simulink model "arinc429_decoder"  (R2021a)
settings: Solver=VariableStepAuto  StartTime=0.0  StopTime=32e-5  RelTol=1e-3
libraries: fl_lib x72, ee_lib x26, nesl_utility x10
(part 1 of 2)
settings Model: Creator=sbetu  LastModifiedBy=sbetu

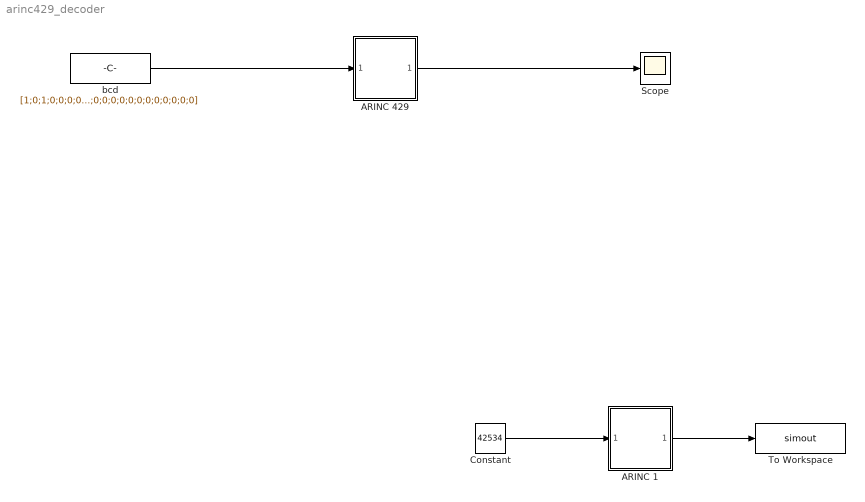
== system arinc429_decoder ==
  ARINC 1 : Subsystem
  ARINC 429 : Subsystem
  Constant : Constant  Value=42534  OutDataTypeStr=double
  Scope : Scope
  To Workspace : ToWorkspace  VariableName=simout  SampleTime=-1
  bcd : Constant  Value=[1;0;1;0;0;0;0;0;0;0;0;0;0;0;0;0;0;0;0]  VectorParams1D=off
  wires:
  bcd/1 -> ARINC 429/1(data 11-29)
  ARINC 429/1(Outport) -> Scope/1
  ARINC 1/1(Outport) -> To Workspace/1
  Constant/1 -> ARINC 1/1(data 11-29)

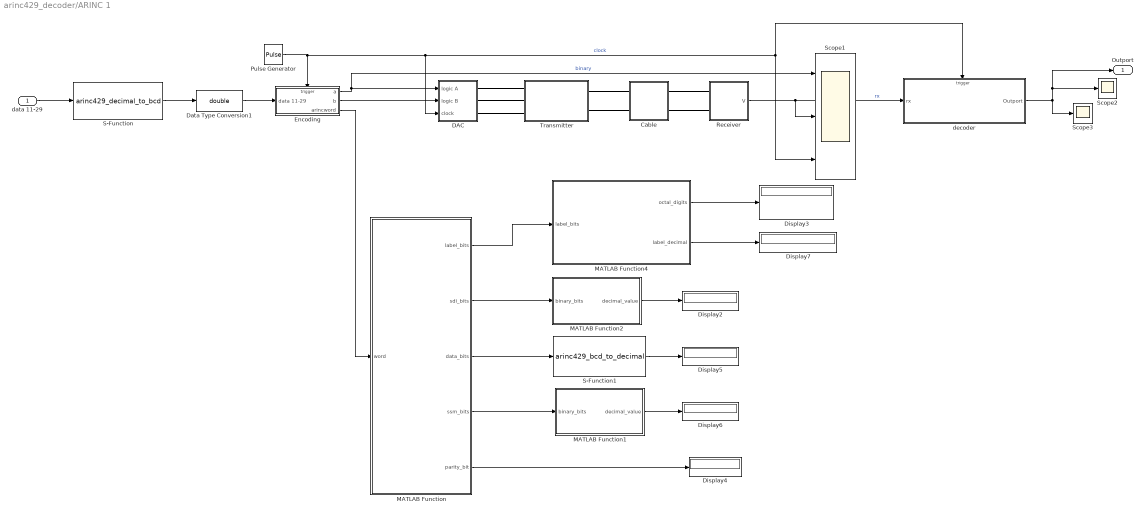
== system arinc429_decoder/ARINC 1 ==
  data 11-29 : Inport
  Cable : Subsystem
  DAC : Subsystem
  Data Type Conversion1 : DataTypeConversion  OutDataTypeStr=double
  Display{2..7} (6 alike) : Display
  Encoding : Subsystem  TreatAsAtomicUnit=on
  MATLAB Function : MATLAB Function  TreatAsAtomicUnit=on
  MATLAB Function1 : MATLAB Function  TreatAsAtomicUnit=on
  MATLAB Function2 : MATLAB Function  TreatAsAtomicUnit=on
  MATLAB Function4 : MATLAB Function  TreatAsAtomicUnit=on
  Pulse Generator : DiscretePulseGenerator  PulseType=Time based  Period=1e-05  PulseWidth=50  PhaseDelay=1e-06
  Receiver : Subsystem
  S-Function : S-Function  FunctionName=arinc429_decimal_to_bcd  SFunctionDeploymentMode=off  EnableBusSupport=off
  S-Function1 : S-Function  FunctionName=arinc429_bcd_to_decimal  SFunctionDeploymentMode=off  EnableBusSupport=off
  Scope1 : Scope  NumInputPorts=3
  Scope2 : Scope
  Scope3 : Scope
  Transmitter : Subsystem
  "decoder " : Subsystem  TreatAsAtomicUnit=on
  Outport : Outport
  wires:
  Encoding/1(a) -> DAC/1(logic A), Scope1/1  "binary"
  Pulse Generator/1 -> Encoding/Trigger, DAC/3(clock), Scope1/3, "decoder "/Trigger  "clock"
  Encoding/2(b) -> DAC/2(logic B)
  "decoder "/1(Outport) -> Outport/1, Scope2/1, Scope3/1
  Receiver/1(V) -> Scope1/2, "decoder "/1(rx)  "rx"
  S-Function/1 -> Data Type Conversion1/1
  Data Type Conversion1/1 -> Encoding/1(data 11-29)
  data 11-29/1 -> S-Function/1
  Encoding/3(arincword) -> MATLAB Function/1(word)
  MATLAB Function/2(sdi_bits) -> MATLAB Function2/1(binary_bits)
  MATLAB Function/4(ssm_bits) -> MATLAB Function1/1(binary_bits)
  MATLAB Function/5(parity_bit) -> Display4/1
  MATLAB Function/3(data_bits) -> S-Function1/1
  S-Function1/1 -> Display5/1
  MATLAB Function2/1(decimal_value) -> Display2/1
  MATLAB Function1/1(decimal_value) -> Display6/1
  MATLAB Function/1(label_bits) -> MATLAB Function4/1(label_bits)
  MATLAB Function4/1(octal_digits) -> Display3/1
  MATLAB Function4/2(label_decimal) -> Display7/1
  connections:
  Cable/LConn1 -- Transmitter/RConn1
  DAC/RConn3 -- Transmitter/LConn3
  DAC/RConn2 -- Transmitter/LConn2
  Cable/LConn2 -- Transmitter/RConn2
  Transmitter/LConn1 -- DAC/RConn1
  Cable/RConn1 -- Receiver/LConn1
  Cable/RConn2 -- Receiver/LConn2

== system arinc429_decoder/ARINC 429 ==
  data 11-29 : Inport
  Cable : Subsystem
  DAC : Subsystem
  Encoding : Subsystem  TreatAsAtomicUnit=on
  Pulse Generator : DiscretePulseGenerator  PulseType=Time based  Period=1e-05  PulseWidth=50  PhaseDelay=1e-06
  Receiver : Subsystem
  Scope1 : Scope  NumInputPorts=3
  Scope3 : Scope
  Transmitter : Subsystem
  "decoder " : Subsystem  TreatAsAtomicUnit=on
  Outport : Outport
  wires:
  Receiver/1(V) -> "decoder "/1(rx), Scope1/2  "rx"
  Encoding/1(a) -> Scope1/1, DAC/1(logic A)  "binary"
  Pulse Generator/1 -> Scope1/3, "decoder "/Trigger, DAC/3(clock), Encoding/Trigger  "clock"
  Encoding/2(b) -> DAC/2(logic B)
  "decoder "/1(Outport) -> Outport/1, Scope3/1
  data 11-29/1 -> Encoding/1(data 11-29)
  connections:
  Cable/LConn1 -- Transmitter/RConn1
  DAC/RConn3 -- Transmitter/LConn3
  DAC/RConn2 -- Transmitter/LConn2
  Cable/LConn2 -- Transmitter/RConn2
  Transmitter/LConn1 -- DAC/RConn1
  Cable/RConn1 -- Receiver/LConn1
  Cable/RConn2 -- Receiver/LConn2

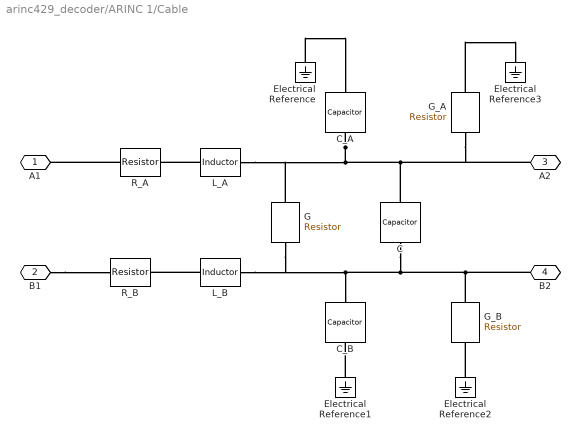
== system arinc429_decoder/ARINC 1/Cable ==
  C : ee_lib/Passive/Capacitor  cap_option=0  c=50e-12 F  Cvec=[1e-05, 1e-06] F  Vvec=[0, 10] V  CV_table_symmetry=1  f_vec=[1, 10] kHz  DFext_vec=[.8, 1.2]  C_tol=5  enable_C_tol=0  tol_distribution=1  nSigma=4  r=0 Ohm  g=0 1/Ohm  averaging_period=0 s  enable_operating_limits=0  operating_limit_action=2  max_working_voltage_range=[-25, 25] V  power_rating=1 W  enable_faults=0  fault_action=1  Cscale_faulted=100  R_faulted=1e-3 Ohm  G_faulted=0 1/Ohm  tau_fault=1e-3 s  enable_temporal_fault=0  t_fault=1 s  enable_behavioral_fault=0  max_permissible_voltage_range=[-100, 100] V  t_fail_on_voltage=1 s  i_specify=off  i_priority=None  i=0 A  i_nominal_specify=off  i_nominal_unit=A  i_nominal_value=1  v_specify=off  v_priority=None  v=0 V  v_nominal_specify=off  v_nominal_unit=V  v_nominal_value=1  vc_specify=off  vc_priority=High  vc=0 V  vc_nominal_specify=off  vc_nominal_unit=V  vc_nominal_value=1
  C_A : ee_lib/Passive/Capacitor  cap_option=0  c=500e-12 F  Cvec=[1e-05, 1e-06] F  Vvec=[0, 10] V  CV_table_symmetry=1  f_vec=[1, 10] kHz  DFext_vec=[.8, 1.2]  C_tol=0  enable_C_tol=0  tol_distribution=1  nSigma=4  r=0 Ohm  g=0 1/Ohm  averaging_period=0 s  enable_operating_limits=0  operating_limit_action=2  max_working_voltage_range=[-25, 25] V  power_rating=1 W  enable_faults=0  fault_action=1  Cscale_faulted=100  R_faulted=1e-3 Ohm  G_faulted=0 1/Ohm  tau_fault=1e-3 s  enable_temporal_fault=0  t_fault=1 s  enable_behavioral_fault=0  max_permissible_voltage_range=[-100, 100] V  t_fail_on_voltage=1 s  i_specify=off  i_priority=None  i=0 A  i_nominal_specify=off  i_nominal_unit=A  i_nominal_value=1  v_specify=off  v_priority=None  v=0 V  v_nominal_specify=off  v_nominal_unit=V  v_nominal_value=1  vc_specify=off  vc_priority=High  vc=0 V  vc_nominal_specify=off  vc_nominal_unit=V  vc_nominal_value=1
  C_B : ee_lib/Passive/Capacitor  cap_option=0  c=500e-12 F  Cvec=[1e-05, 1e-06] F  Vvec=[0, 10] V  CV_table_symmetry=1  f_vec=[1, 10] kHz  DFext_vec=[.8, 1.2]  C_tol=0  enable_C_tol=0  tol_distribution=1  nSigma=4  r=0 Ohm  g=0 1/Ohm  averaging_period=0 s  enable_operating_limits=0  operating_limit_action=2  max_working_voltage_range=[-25, 25] V  power_rating=1 W  enable_faults=0  fault_action=1  Cscale_faulted=100  R_faulted=1e-3 Ohm  G_faulted=0 1/Ohm  tau_fault=1e-3 s  enable_temporal_fault=0  t_fault=1 s  enable_behavioral_fault=0  max_permissible_voltage_range=[-100, 100] V  t_fail_on_voltage=1 s  i_specify=off  i_priority=None  i=0 A  i_nominal_specify=off  i_nominal_unit=A  i_nominal_value=1  v_specify=off  v_priority=None  v=0 V  v_nominal_specify=off  v_nominal_unit=V  v_nominal_value=1  vc_specify=off  vc_priority=High  vc=0 V  vc_nominal_specify=off  vc_nominal_unit=V  vc_nominal_value=1
  Electrical Reference{,1..3} (4 alike) : fl_lib/Electrical/Electrical Elements/Electrical Reference
  G : fl_lib/Electrical/Electrical Elements/Resistor  R=1 MOhm  i_specify=off  i_priority=None  i=0 A  i_nominal_specify=off  i_nominal_unit=A  i_nominal_value=1  v_specify=off  v_priority=None  v=0 V  v_nominal_specify=off  v_nominal_unit=V  v_nominal_value=1
  G_A : fl_lib/Electrical/Electrical Elements/Resistor  R=100 MOhm  i_specify=off  i_priority=None  i=0 A  i_nominal_specify=off  i_nominal_unit=A  i_nominal_value=1  v_specify=off  v_priority=None  v=0 V  v_nominal_specify=off  v_nominal_unit=V  v_nominal_value=1
  G_B : fl_lib/Electrical/Electrical Elements/Resistor  R=100 MOhm  i_specify=off  i_priority=None  i=0 A  i_nominal_specify=off  i_nominal_unit=A  i_nominal_value=1  v_specify=off  v_priority=None  v=0 V  v_nominal_specify=off  v_nominal_unit=V  v_nominal_value=1
  L_A : ee_lib/Passive/Inductor  l=5 mH  L_tol=0  enable_L_tol=0  tol_distribution=1  nSigma=4  r=0 Ohm  g=1e-9 S  enable_operating_limits=0  operating_limit_action=2  max_working_current=1 A  power_rating=1 W  enable_faults=0  fault_action=1  lambdaPercent=50  k_faulted=0.9999  turnsShort=0  openCct=0  groundShort=0  groundShortG=0 1/Ohm  tau_fault=1e-3 s  enable_temporal_fault=0  t_fault=1 s  enable_behavioral_fault=0  max_permissible_voltage=100 V  n_fail_on_voltage=1  max_permissible_current=1 A  t_fail_on_current=1 s  i_L_specify=off  i_L_priority=High  i_L=0 A  i_L_nominal_specify=off  i_L_nominal_unit=A  i_L_nominal_value=1
  L_B : ee_lib/Passive/Inductor  l=5 mH  L_tol=0  enable_L_tol=0  tol_distribution=1  nSigma=4  r=0 Ohm  g=1e-9 S  enable_operating_limits=0  operating_limit_action=2  max_working_current=1 A  power_rating=1 W  enable_faults=0  fault_action=1  lambdaPercent=50  k_faulted=0.9999  turnsShort=0  openCct=0  groundShort=0  groundShortG=0 1/Ohm  tau_fault=1e-3 s  enable_temporal_fault=0  t_fault=1 s  enable_behavioral_fault=0  max_permissible_voltage=100 V  n_fail_on_voltage=1  max_permissible_current=1 A  t_fail_on_current=1 s  i_L_specify=off  i_L_priority=High  i_L=0 A  i_L_nominal_specify=off  i_L_nominal_unit=A  i_L_nominal_value=1
  R_A : fl_lib/Electrical/Electrical Elements/Resistor  R=0.65 Ohm  i_specify=off  i_priority=None  i=0 A  i_nominal_specify=off  i_nominal_unit=A  i_nominal_value=1  v_specify=off  v_priority=None  v=0 V  v_nominal_specify=off  v_nominal_unit=V  v_nominal_value=1
  R_B : fl_lib/Electrical/Electrical Elements/Resistor  R=0.65 Ohm  i_specify=off  i_priority=None  i=0 A  i_nominal_specify=off  i_nominal_unit=A  i_nominal_value=1  v_specify=off  v_priority=None  v=0 V  v_nominal_specify=off  v_nominal_unit=V  v_nominal_value=1
  A1 : PMIOPort  Side=Left
  B1 : PMIOPort  Port=2  Side=Left
  A2 : PMIOPort  Port=3  Side=Right
  B2 : PMIOPort  Port=4  Side=Right
  connections:
  C_A/RConn1 -- G/LConn1 -- L_A/RConn1 -- G_A/RConn1 -- A2/RConn1 -- C/LConn1
  B2/RConn1 -- G_B/LConn1 -- C/RConn1 -- L_B/RConn1 -- G/RConn1 -- C_B/LConn1
  L_A/LConn1 -- R_A/RConn1
  Electrical Reference1/LConn1 -- C_B/RConn1
  L_B/LConn1 -- R_B/RConn1
  R_A/LConn1 -- A1/RConn1
  G_A/LConn1 -- Electrical Reference3/LConn1
  Electrical Reference2/LConn1 -- G_B/RConn1
  Electrical Reference/LConn1 -- C_A/LConn1
  B1/RConn1 -- R_B/LConn1

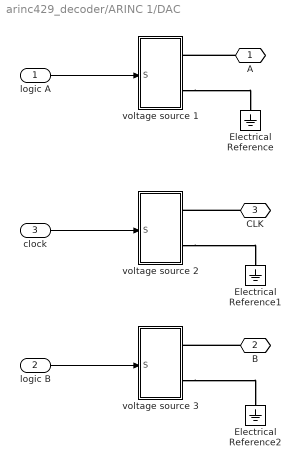
== system arinc429_decoder/ARINC 1/DAC ==
  logic A : Inport
  logic B : Inport  Port=2
  clock : Inport  Port=3
  Electrical Reference : fl_lib/Electrical/Electrical Elements/Electrical Reference
  Electrical Reference1 : fl_lib/Electrical/Electrical Elements/Electrical Reference
  Electrical Reference2 : fl_lib/Electrical/Electrical Elements/Electrical Reference
  voltage source 1 : Subsystem
  voltage source 2 : Subsystem
  voltage source 3 : Subsystem
  A : PMIOPort  Side=Right
  B : PMIOPort  Port=2  Side=Right
  CLK : PMIOPort  Port=3  Side=Right
  wires:
  logic A/1 -> voltage source 1/1(S)
  logic B/1 -> voltage source 3/1(S)
  clock/1 -> voltage source 2/1(S)
  connections:
  voltage source 1/RConn2 -- Electrical Reference/LConn1
  voltage source 3/RConn2 -- Electrical Reference2/LConn1
  CLK/RConn1 -- voltage source 2/RConn1
  voltage source 2/RConn2 -- Electrical Reference1/LConn1
  B/RConn1 -- voltage source 3/RConn1
  A/RConn1 -- voltage source 1/RConn1

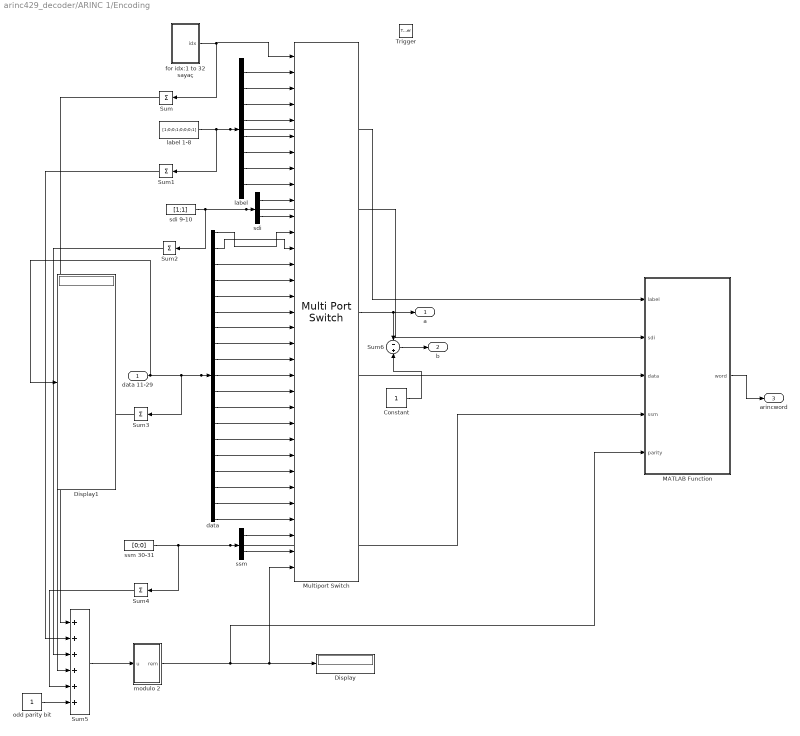
== system arinc429_decoder/ARINC 1/Encoding ==
  data 11-29 : Inport
  Trigger : TriggerPort  VariantControl=(inherit)
  Constant : Constant
  Display : Display
  Display1 : Display
  MATLAB Function : MATLAB Function  TreatAsAtomicUnit=on
  Multiport Switch : MultiPortSwitch  Inputs=32  DiagnosticForDefault=None  InputSameDT=on
  Sum{,1..4} (5 alike) : Sum  Inputs=+
  Sum5 : Sum  Inputs=++++++
  Sum6 : Sum  Inputs=-+
  data : Demux  Outputs=19
  for idx:1 to 32 sayaç : Subsystem
  label : Demux  Outputs=8
  label 1-8 : Constant  Value=[1;0;0;1;0;0;0;1]  VectorParams1D=off
  modulo 2 : Subsystem
  odd parity bit : Constant
  sdi : Demux  Outputs=2
  sdi 9-10 : Constant  Value=[1;1]  VectorParams1D=off
  ssm : Demux  Outputs=2
  ssm 30-31 : Constant  Value=[0;0]  VectorParams1D=off
  a : Outport
  b : Outport  Port=2
  arincword : Outport  Port=3
  wires:
  for idx:1 to 32 sayaç/1(idx) -> Sum/1, Multiport Switch/1
  label/8 -> Multiport Switch/9
  label/7 -> Multiport Switch/8
  label/6 -> Multiport Switch/7
  label/5 -> Multiport Switch/6
  label/4 -> Multiport Switch/5
  label/3 -> Multiport Switch/4
  label/2 -> Multiport Switch/3
  label 1-8/1 -> Sum1/1, MATLAB Function/1(label), label/1
  sdi/1 -> Multiport Switch/10
  sdi/2 -> Multiport Switch/11
  sdi 9-10/1 -> Sum2/1, MATLAB Function/2(sdi), sdi/1
  data/19 -> Multiport Switch/30
  data/18 -> Multiport Switch/29
  data/17 -> Multiport Switch/28
  data/16 -> Multiport Switch/27
  data/15 -> Multiport Switch/26
  data/14 -> Multiport Switch/25
  data/13 -> Multiport Switch/24
  data/12 -> Multiport Switch/23
  data/11 -> Multiport Switch/22
  data/10 -> Multiport Switch/21
  data/9 -> Multiport Switch/20
  data/8 -> Multiport Switch/19
  data/7 -> Multiport Switch/18
  data/6 -> Multiport Switch/17
  data/5 -> Multiport Switch/16
  data/4 -> Multiport Switch/15
  data/3 -> Multiport Switch/14
  data/2 -> Multiport Switch/13
  data/1 -> Multiport Switch/12
  data 11-29/1 -> Sum3/1, MATLAB Function/3(data), data/1, Display1/1
  ssm/1 -> Multiport Switch/31
  ssm/2 -> Multiport Switch/32
  ssm 30-31/1 -> Sum4/1, MATLAB Function/4(ssm), ssm/1
  Sum5/1 -> modulo 2/1(u)
  Sum/1 -> Sum5/1
  Sum1/1 -> Sum5/2
  Sum2/1 -> Sum5/3
  Sum3/1 -> Sum5/4
  Sum4/1 -> Sum5/5
  odd parity bit/1 -> Sum5/6
  Multiport Switch/1 -> Sum6/1, a/1
  Constant/1 -> Sum6/2
  Sum6/1 -> b/1
  modulo 2/1(rem) -> MATLAB Function/5(parity), Display/1, Multiport Switch/33
  label/1 -> Multiport Switch/2
  MATLAB Function/1(word) -> arincword/1

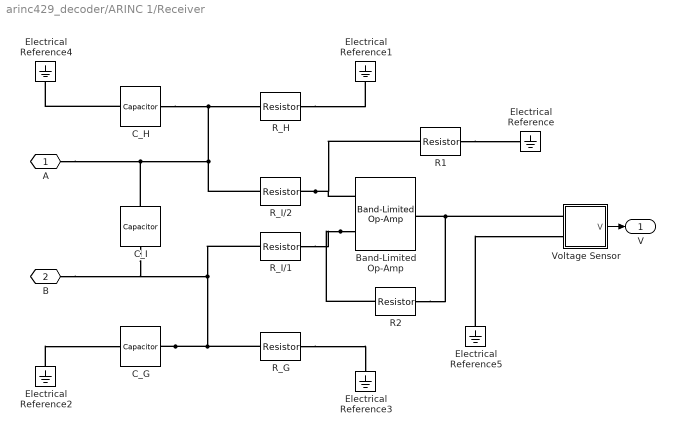
== system arinc429_decoder/ARINC 1/Receiver ==
  Band-Limited Op-Amp : ee_lib/Integrated Circuits/Band-Limited Op-Amp  A=1000  Rin=1e6 Ohm  Rout=100 Ohm  Vmin=-10 V  Vmax=10 V  Vdotmax=1e7 V/s  f=1e6 Hz  V0=0 V
      settings: SourceProductBaseCode=PS
  C_G : ee_lib/Passive/Capacitor  cap_option=0  c=50e-12 F  Cvec=[1e-05, 1e-06] F  Vvec=[0, 10] V  CV_table_symmetry=1  f_vec=[1, 10] kHz  DFext_vec=[.8, 1.2]  C_tol=0  enable_C_tol=0  tol_distribution=1  nSigma=4  r=1e-6 Ohm  g=0 1/Ohm  averaging_period=0 s  enable_operating_limits=0  operating_limit_action=2  max_working_voltage_range=[-25, 25] V  power_rating=1 W  enable_faults=0  fault_action=1  Cscale_faulted=100  R_faulted=1e-3 Ohm  G_faulted=0 1/Ohm  tau_fault=1e-3 s  enable_temporal_fault=0  t_fault=1 s  enable_behavioral_fault=0  max_permissible_voltage_range=[-100, 100] V  t_fail_on_voltage=1 s  i_specify=off  i_priority=None  i=0 A  i_nominal_specify=off  i_nominal_unit=A  i_nominal_value=1  v_specify=off  v_priority=None  v=0 V  v_nominal_specify=off  v_nominal_unit=V  v_nominal_value=1  vc_specify=off  vc_priority=High  vc=0 V  vc_nominal_specify=off  vc_nominal_unit=V  vc_nominal_value=1
  C_H : ee_lib/Passive/Capacitor  cap_option=0  c=50e-12 F  Cvec=[1e-05, 1e-06] F  Vvec=[0, 10] V  CV_table_symmetry=1  f_vec=[1, 10] kHz  DFext_vec=[.8, 1.2]  C_tol=0  enable_C_tol=0  tol_distribution=1  nSigma=4  r=1e-6 Ohm  g=0 1/Ohm  averaging_period=0 s  enable_operating_limits=0  operating_limit_action=2  max_working_voltage_range=[-25, 25] V  power_rating=1 W  enable_faults=0  fault_action=1  Cscale_faulted=100  R_faulted=1e-3 Ohm  G_faulted=0 1/Ohm  tau_fault=1e-3 s  enable_temporal_fault=0  t_fault=1 s  enable_behavioral_fault=0  max_permissible_voltage_range=[-100, 100] V  t_fail_on_voltage=1 s  i_specify=off  i_priority=None  i=0 A  i_nominal_specify=off  i_nominal_unit=A  i_nominal_value=1  v_specify=off  v_priority=None  v=0 V  v_nominal_specify=off  v_nominal_unit=V  v_nominal_value=1  vc_specify=off  vc_priority=High  vc=0 V  vc_nominal_specify=off  vc_nominal_unit=V  vc_nominal_value=1
  C_I : ee_lib/Passive/Capacitor  cap_option=0  c=50e-12 F  Cvec=[1e-05, 1e-06] F  Vvec=[0, 10] V  CV_table_symmetry=1  f_vec=[1, 10] kHz  DFext_vec=[.8, 1.2]  C_tol=0  enable_C_tol=0  tol_distribution=1  nSigma=4  r=1e-6 Ohm  g=0 1/Ohm  averaging_period=0 s  enable_operating_limits=0  operating_limit_action=2  max_working_voltage_range=[-25, 25] V  power_rating=1 W  enable_faults=0  fault_action=1  Cscale_faulted=100  R_faulted=1e-3 Ohm  G_faulted=0 1/Ohm  tau_fault=1e-3 s  enable_temporal_fault=0  t_fault=1 s  enable_behavioral_fault=0  max_permissible_voltage_range=[-100, 100] V  t_fail_on_voltage=1 s  i_specify=off  i_priority=None  i=0 A  i_nominal_specify=off  i_nominal_unit=A  i_nominal_value=1  v_specify=off  v_priority=None  v=0 V  v_nominal_specify=off  v_nominal_unit=V  v_nominal_value=1  vc_specify=off  vc_priority=High  vc=0 V  vc_nominal_specify=off  vc_nominal_unit=V  vc_nominal_value=1
  Electrical Reference{,1..5} (6 alike) : fl_lib/Electrical/Electrical Elements/Electrical Reference
  R1 : fl_lib/Electrical/Electrical Elements/Resistor  R=6 kOhm  i_specify=off  i_priority=None  i=0 A  i_nominal_specify=off  i_nominal_unit=A  i_nominal_value=1  v_specify=off  v_priority=None  v=0 V  v_nominal_specify=off  v_nominal_unit=V  v_nominal_value=1
  R2 : fl_lib/Electrical/Electrical Elements/Resistor  R=6 kOhm  i_specify=off  i_priority=None  i=0 A  i_nominal_specify=off  i_nominal_unit=A  i_nominal_value=1  v_specify=off  v_priority=None  v=0 V  v_nominal_specify=off  v_nominal_unit=V  v_nominal_value=1
  R_G : fl_lib/Electrical/Electrical Elements/Resistor  R=12 kOhm  i_specify=off  i_priority=None  i=0 A  i_nominal_specify=off  i_nominal_unit=A  i_nominal_value=1  v_specify=off  v_priority=None  v=0 V  v_nominal_specify=off  v_nominal_unit=V  v_nominal_value=1
  R_H : fl_lib/Electrical/Electrical Elements/Resistor  R=12 kOhm  i_specify=off  i_priority=None  i=0 A  i_nominal_specify=off  i_nominal_unit=A  i_nominal_value=1  v_specify=off  v_priority=None  v=0 V  v_nominal_specify=off  v_nominal_unit=V  v_nominal_value=1
  R_I/1 : fl_lib/Electrical/Electrical Elements/Resistor  R=12 kOhm  i_specify=off  i_priority=None  i=0 A  i_nominal_specify=off  i_nominal_unit=A  i_nominal_value=1  v_specify=off  v_priority=None  v=0 V  v_nominal_specify=off  v_nominal_unit=V  v_nominal_value=1
  R_I/2 : fl_lib/Electrical/Electrical Elements/Resistor  R=12 kOhm  i_specify=off  i_priority=None  i=0 A  i_nominal_specify=off  i_nominal_unit=A  i_nominal_value=1  v_specify=off  v_priority=None  v=0 V  v_nominal_specify=off  v_nominal_unit=V  v_nominal_value=1
  Voltage Sensor : Subsystem
  A : PMIOPort  Side=Left
  B : PMIOPort  Port=2  Side=Left
  V : Outport
  wires:
  Voltage Sensor/1(V) -> V/1
  connections:
  R1/RConn1 -- Electrical Reference/LConn1
  C_G/LConn1 -- R_G/LConn1 -- B/RConn1 -- C_I/RConn1 -- R_I/1/LConn1
  C_I/LConn1 -- A/RConn1 -- R_I/2/LConn1 -- C_H/LConn1 -- R_H/LConn1
  Band-Limited Op-Amp/LConn2 -- R_I/1/RConn1 -- R2/LConn1
  R_I/2/RConn1 -- R1/LConn1 -- Band-Limited Op-Amp/LConn1
  Electrical Reference2/LConn1 -- C_G/RConn1
  R_H/RConn1 -- Electrical Reference1/LConn1
  Electrical Reference5/LConn1 -- Voltage Sensor/LConn2
  R_G/RConn1 -- Electrical Reference3/LConn1
  C_H/RConn1 -- Electrical Reference4/LConn1
  R2/RConn1 -- Band-Limited Op-Amp/RConn1 -- Voltage Sensor/LConn1

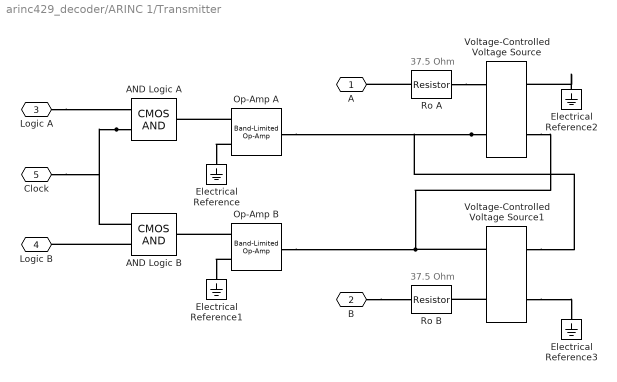
== system arinc429_decoder/ARINC 1/Transmitter ==
  note: 37.5 Ohm
  note: 37.5 Ohm
  " Op-Amp A" : ee_lib/Integrated Circuits/Band-Limited Op-Amp  A=1000  Rin=1e6 Ohm  Rout=37.5 Ohm  Vmin=-15 V  Vmax=15 V  Vdotmax=2e7 V/s  f=1e6 Hz  V0=0 V
      settings: SourceProductBaseCode=PS
  " Op-Amp B" : ee_lib/Integrated Circuits/Band-Limited Op-Amp  A=1000  Rin=1e6 Ohm  Rout=37.5 Ohm  Vmin=-10 V  Vmax=10 V  Vdotmax=2e7 V/s  f=1e6 Hz  V0=0 V
      settings: SourceProductBaseCode=PS
  AND Logic A : ee_lib/Integrated Circuits/Logic/CMOS AND  V_IL=0.1 V  V_IH=5 V  C_IN=5 pF  output_type=1  V_OL=0 V  V_OH=6.5 V  V_CC=5 V  V_meas=5 V  R_OUT=37.5 Ohm  R_OH=[25, 250] Ohm  I_OH=63 mA  R_OL=[30, 800] Ohm  I_OL=-45 mA  Delay=25 ns  Ron=5 Ohm  Vf=0.6 V  output_state=1
      settings: SourceProductBaseCode=PS  InternalSimscapePortConfiguration="{\"Bottom\":[],\"Left\":[{\"id\":\"A\",\"label\":\"\",\"type\":\"foundation.electrical.electrical\"},{\"id\":\"B\",\"label\":\"\",\"type\":\"foundation.electrical.electrical\"}],\"Right\":[{\"id\":\"J\",\"label\":\"\",\"type\":\"foundation.electrical.electrical\"}],\"Top\":[]}"
  AND Logic B : ee_lib/Integrated Circuits/Logic/CMOS AND  V_IL=0.1 V  V_IH=5 V  C_IN=5 pF  output_type=1  V_OL=0 V  V_OH=6.5 V  V_CC=5 V  V_meas=5 V  R_OUT=37.5 Ohm  R_OH=[25, 250] Ohm  I_OH=63 mA  R_OL=[30, 800] Ohm  I_OL=-45 mA  Delay=25 ns  Ron=5 Ohm  Vf=0.6 V  output_state=1
      settings: SourceProductBaseCode=PS  InternalSimscapePortConfiguration="{\"Bottom\":[],\"Left\":[{\"id\":\"A\",\"label\":\"\",\"type\":\"foundation.electrical.electrical\"},{\"id\":\"B\",\"label\":\"\",\"type\":\"foundation.electrical.electrical\"}],\"Right\":[{\"id\":\"J\",\"label\":\"\",\"type\":\"foundation.electrical.electrical\"}],\"Top\":[]}"
  Electrical Reference{,1..3} (4 alike) : fl_lib/Electrical/Electrical Elements/Electrical Reference
  Ro A : fl_lib/Electrical/Electrical Elements/Resistor  R=37.5 Ohm  i_specify=off  i_priority=None  i=0 A  i_nominal_specify=off  i_nominal_unit=A  i_nominal_value=1  v_specify=off  v_priority=None  v=0 V  v_nominal_specify=off  v_nominal_unit=V  v_nominal_value=1
  Ro B : fl_lib/Electrical/Electrical Elements/Resistor  R=37.5 Ohm  i_specify=off  i_priority=None  i=0 A  i_nominal_specify=off  i_nominal_unit=A  i_nominal_value=1  v_specify=off  v_priority=None  v=0 V  v_nominal_specify=off  v_nominal_unit=V  v_nominal_value=1
  Voltage-Controlled Voltage Source : fl_lib/Electrical/Electrical Sources/Voltage-Controlled Voltage Source  K=2.5  v1_specify=off  v1_priority=None  v1=0 V  v1_nominal_specify=off  v1_nominal_unit=V  v1_nominal_value=1  v2_specify=off  v2_priority=None  v2=0 V  v2_nominal_specify=off  v2_nominal_unit=V  v2_nominal_value=1
      settings: SourceProductBaseCode=SS  InternalSimscapePortConfiguration="{\"Bottom\":[],\"Left\":[{\"id\":\"p1\",\"label\":\"+\",\"type\":\"foundation.electrical.electrical\"},{\"id\":\"p2\",\"label\":\"+\",\"type\":\"foundation.electrical.electrical\"}],\"Right\":[{\"id\":\"n1\",\"label\":\"-\",\"type\":\"foundation.electrical.electrical\"},{\"id\":\"n2\",\"label\":\"-\",\"type\":\"foundation.electrical.electrical\"}],\"Top\":[]}"
  Voltage-Controlled Voltage Source1 : fl_lib/Electrical/Electrical Sources/Voltage-Controlled Voltage Source  K=2.5  v1_specify=off  v1_priority=None  v1=0 V  v1_nominal_specify=off  v1_nominal_unit=V  v1_nominal_value=1  v2_specify=off  v2_priority=None  v2=0 V  v2_nominal_specify=off  v2_nominal_unit=V  v2_nominal_value=1
      settings: SourceProductBaseCode=SS  InternalSimscapePortConfiguration="{\"Bottom\":[],\"Left\":[{\"id\":\"p1\",\"label\":\"+\",\"type\":\"foundation.electrical.electrical\"},{\"id\":\"p2\",\"label\":\"+\",\"type\":\"foundation.electrical.electrical\"}],\"Right\":[{\"id\":\"n1\",\"label\":\"-\",\"type\":\"foundation.electrical.electrical\"},{\"id\":\"n2\",\"label\":\"-\",\"type\":\"foundation.electrical.electrical\"}],\"Top\":[]}"
  A : PMIOPort  Side=Right
  B : PMIOPort  Port=2  Side=Right
  Logic A : PMIOPort  Port=3  Side=Left
  Logic B : PMIOPort  Port=4  Side=Left
  Clock : PMIOPort  Port=5  Side=Left
  connections:
  Voltage-Controlled Voltage Source/RConn1 -- " Op-Amp B"/RConn1 -- Voltage-Controlled Voltage Source1/LConn1
  Voltage-Controlled Voltage Source/LConn1 -- " Op-Amp A"/RConn1 -- Voltage-Controlled Voltage Source1/RConn1
  AND Logic A/LConn2 -- Clock/RConn1 -- AND Logic B/LConn1
  " Op-Amp A"/LConn1 -- AND Logic A/RConn1
  " Op-Amp B"/LConn1 -- AND Logic B/RConn1
  Electrical Reference2/LConn1 -- Voltage-Controlled Voltage Source/RConn2
  AND Logic B/LConn2 -- Logic B/RConn1
  Ro A/LConn1 -- Voltage-Controlled Voltage Source/LConn2
  " Op-Amp A"/LConn2 -- Electrical Reference/LConn1
  Voltage-Controlled Voltage Source1/RConn2 -- Electrical Reference3/LConn1
  Ro A/RConn1 -- A/RConn1
  Logic A/RConn1 -- AND Logic A/LConn1
  " Op-Amp B"/LConn2 -- Electrical Reference1/LConn1
  Voltage-Controlled Voltage Source1/LConn2 -- Ro B/LConn1
  B/RConn1 -- Ro B/RConn1

== system arinc429_decoder/ARINC 1/decoder  ==
  rx : Inport
  Trigger : TriggerPort  VariantControl=(inherit)
  Constant : Constant  Value=5
  Constant1 : Constant  Value=-5
  Constant2 : Constant  Value=0
  Relational Operator : RelationalOperator  Operator=>  OutDataTypeStr=boolean  RndMeth=Simplest
  Relational Operator1 : RelationalOperator  Operator=<  OutDataTypeStr=boolean  RndMeth=Simplest
  Switch : Switch  Criteria=u2 ~= 0
  Outport : Outport
  wires:
  Constant1/1 -> Relational Operator1/1
  Constant/1 -> Relational Operator/1
  Constant2/1 -> Switch/2
  Relational Operator1/1 -> Switch/3
  Relational Operator/1 -> Switch/1
  Switch/1 -> Outport/1
  rx/1 -> Relational Operator1/2, Relational Operator/2

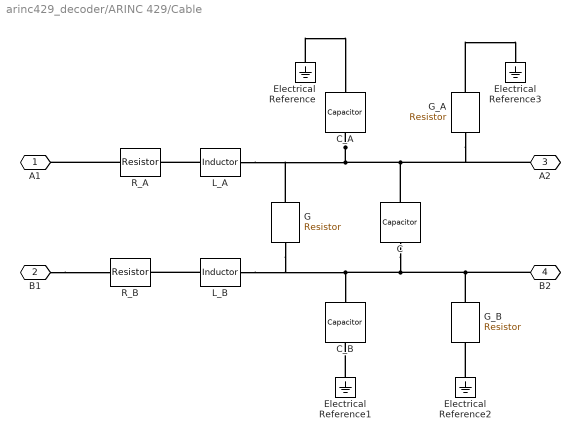
== system arinc429_decoder/ARINC 429/Cable ==
  C : ee_lib/Passive/Capacitor  cap_option=0  c=50e-12 F  Cvec=[1e-05, 1e-06] F  Vvec=[0, 10] V  CV_table_symmetry=1  f_vec=[1, 10] kHz  DFext_vec=[.8, 1.2]  C_tol=5  enable_C_tol=0  tol_distribution=1  nSigma=4  r=0 Ohm  g=0 1/Ohm  averaging_period=0 s  enable_operating_limits=0  operating_limit_action=2  max_working_voltage_range=[-25, 25] V  power_rating=1 W  enable_faults=0  fault_action=1  Cscale_faulted=100  R_faulted=1e-3 Ohm  G_faulted=0 1/Ohm  tau_fault=1e-3 s  enable_temporal_fault=0  t_fault=1 s  enable_behavioral_fault=0  max_permissible_voltage_range=[-100, 100] V  t_fail_on_voltage=1 s  i_specify=off  i_priority=None  i=0 A  i_nominal_specify=off  i_nominal_unit=A  i_nominal_value=1  v_specify=off  v_priority=None  v=0 V  v_nominal_specify=off  v_nominal_unit=V  v_nominal_value=1  vc_specify=off  vc_priority=High  vc=0 V  vc_nominal_specify=off  vc_nominal_unit=V  vc_nominal_value=1
  C_A : ee_lib/Passive/Capacitor  cap_option=0  c=500e-12 F  Cvec=[1e-05, 1e-06] F  Vvec=[0, 10] V  CV_table_symmetry=1  f_vec=[1, 10] kHz  DFext_vec=[.8, 1.2]  C_tol=0  enable_C_tol=0  tol_distribution=1  nSigma=4  r=0 Ohm  g=0 1/Ohm  averaging_period=0 s  enable_operating_limits=0  operating_limit_action=2  max_working_voltage_range=[-25, 25] V  power_rating=1 W  enable_faults=0  fault_action=1  Cscale_faulted=100  R_faulted=1e-3 Ohm  G_faulted=0 1/Ohm  tau_fault=1e-3 s  enable_temporal_fault=0  t_fault=1 s  enable_behavioral_fault=0  max_permissible_voltage_range=[-100, 100] V  t_fail_on_voltage=1 s  i_specify=off  i_priority=None  i=0 A  i_nominal_specify=off  i_nominal_unit=A  i_nominal_value=1  v_specify=off  v_priority=None  v=0 V  v_nominal_specify=off  v_nominal_unit=V  v_nominal_value=1  vc_specify=off  vc_priority=High  vc=0 V  vc_nominal_specify=off  vc_nominal_unit=V  vc_nominal_value=1
  C_B : ee_lib/Passive/Capacitor  cap_option=0  c=500e-12 F  Cvec=[1e-05, 1e-06] F  Vvec=[0, 10] V  CV_table_symmetry=1  f_vec=[1, 10] kHz  DFext_vec=[.8, 1.2]  C_tol=0  enable_C_tol=0  tol_distribution=1  nSigma=4  r=0 Ohm  g=0 1/Ohm  averaging_period=0 s  enable_operating_limits=0  operating_limit_action=2  max_working_voltage_range=[-25, 25] V  power_rating=1 W  enable_faults=0  fault_action=1  Cscale_faulted=100  R_faulted=1e-3 Ohm  G_faulted=0 1/Ohm  tau_fault=1e-3 s  enable_temporal_fault=0  t_fault=1 s  enable_behavioral_fault=0  max_permissible_voltage_range=[-100, 100] V  t_fail_on_voltage=1 s  i_specify=off  i_priority=None  i=0 A  i_nominal_specify=off  i_nominal_unit=A  i_nominal_value=1  v_specify=off  v_priority=None  v=0 V  v_nominal_specify=off  v_nominal_unit=V  v_nominal_value=1  vc_specify=off  vc_priority=High  vc=0 V  vc_nominal_specify=off  vc_nominal_unit=V  vc_nominal_value=1
  Electrical Reference{,1..3} (4 alike) : fl_lib/Electrical/Electrical Elements/Electrical Reference
  G : fl_lib/Electrical/Electrical Elements/Resistor  R=1 MOhm  i_specify=off  i_priority=None  i=0 A  i_nominal_specify=off  i_nominal_unit=A  i_nominal_value=1  v_specify=off  v_priority=None  v=0 V  v_nominal_specify=off  v_nominal_unit=V  v_nominal_value=1
  G_A : fl_lib/Electrical/Electrical Elements/Resistor  R=100 MOhm  i_specify=off  i_priority=None  i=0 A  i_nominal_specify=off  i_nominal_unit=A  i_nominal_value=1  v_specify=off  v_priority=None  v=0 V  v_nominal_specify=off  v_nominal_unit=V  v_nominal_value=1
  G_B : fl_lib/Electrical/Electrical Elements/Resistor  R=100 MOhm  i_specify=off  i_priority=None  i=0 A  i_nominal_specify=off  i_nominal_unit=A  i_nominal_value=1  v_specify=off  v_priority=None  v=0 V  v_nominal_specify=off  v_nominal_unit=V  v_nominal_value=1
  L_A : ee_lib/Passive/Inductor  l=5 mH  L_tol=0  enable_L_tol=0  tol_distribution=1  nSigma=4  r=0 Ohm  g=1e-9 S  enable_operating_limits=0  operating_limit_action=2  max_working_current=1 A  power_rating=1 W  enable_faults=0  fault_action=1  lambdaPercent=50  k_faulted=0.9999  turnsShort=0  openCct=0  groundShort=0  groundShortG=0 1/Ohm  tau_fault=1e-3 s  enable_temporal_fault=0  t_fault=1 s  enable_behavioral_fault=0  max_permissible_voltage=100 V  n_fail_on_voltage=1  max_permissible_current=1 A  t_fail_on_current=1 s  i_L_specify=off  i_L_priority=High  i_L=0 A  i_L_nominal_specify=off  i_L_nominal_unit=A  i_L_nominal_value=1
  L_B : ee_lib/Passive/Inductor  l=5 mH  L_tol=0  enable_L_tol=0  tol_distribution=1  nSigma=4  r=0 Ohm  g=1e-9 S  enable_operating_limits=0  operating_limit_action=2  max_working_current=1 A  power_rating=1 W  enable_faults=0  fault_action=1  lambdaPercent=50  k_faulted=0.9999  turnsShort=0  openCct=0  groundShort=0  groundShortG=0 1/Ohm  tau_fault=1e-3 s  enable_temporal_fault=0  t_fault=1 s  enable_behavioral_fault=0  max_permissible_voltage=100 V  n_fail_on_voltage=1  max_permissible_current=1 A  t_fail_on_current=1 s  i_L_specify=off  i_L_priority=High  i_L=0 A  i_L_nominal_specify=off  i_L_nominal_unit=A  i_L_nominal_value=1
  R_A : fl_lib/Electrical/Electrical Elements/Resistor  R=0.65 Ohm  i_specify=off  i_priority=None  i=0 A  i_nominal_specify=off  i_nominal_unit=A  i_nominal_value=1  v_specify=off  v_priority=None  v=0 V  v_nominal_specify=off  v_nominal_unit=V  v_nominal_value=1
  R_B : fl_lib/Electrical/Electrical Elements/Resistor  R=0.65 Ohm  i_specify=off  i_priority=None  i=0 A  i_nominal_specify=off  i_nominal_unit=A  i_nominal_value=1  v_specify=off  v_priority=None  v=0 V  v_nominal_specify=off  v_nominal_unit=V  v_nominal_value=1
  A1 : PMIOPort  Side=Left
  B1 : PMIOPort  Port=2  Side=Left
  A2 : PMIOPort  Port=3  Side=Right
  B2 : PMIOPort  Port=4  Side=Right
  connections:
  C_A/RConn1 -- G/LConn1 -- L_A/RConn1 -- G_A/RConn1 -- A2/RConn1 -- C/LConn1
  B2/RConn1 -- G_B/LConn1 -- C/RConn1 -- L_B/RConn1 -- G/RConn1 -- C_B/LConn1
  L_A/LConn1 -- R_A/RConn1
  Electrical Reference1/LConn1 -- C_B/RConn1
  L_B/LConn1 -- R_B/RConn1
  R_A/LConn1 -- A1/RConn1
  G_A/LConn1 -- Electrical Reference3/LConn1
  Electrical Reference2/LConn1 -- G_B/RConn1
  Electrical Reference/LConn1 -- C_A/LConn1
  B1/RConn1 -- R_B/LConn1

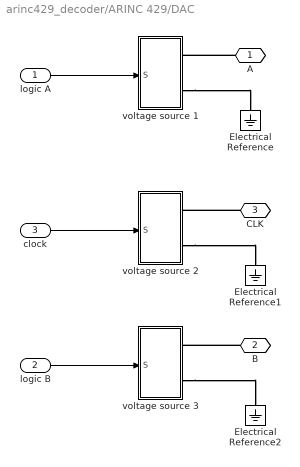
== system arinc429_decoder/ARINC 429/DAC ==
  logic A : Inport
  logic B : Inport  Port=2
  clock : Inport  Port=3
  Electrical Reference : fl_lib/Electrical/Electrical Elements/Electrical Reference
  Electrical Reference1 : fl_lib/Electrical/Electrical Elements/Electrical Reference
  Electrical Reference2 : fl_lib/Electrical/Electrical Elements/Electrical Reference
  voltage source 1 : Subsystem
  voltage source 2 : Subsystem
  voltage source 3 : Subsystem
  A : PMIOPort  Side=Right
  B : PMIOPort  Port=2  Side=Right
  CLK : PMIOPort  Port=3  Side=Right
  wires:
  logic A/1 -> voltage source 1/1(S)
  logic B/1 -> voltage source 3/1(S)
  clock/1 -> voltage source 2/1(S)
  connections:
  voltage source 1/RConn2 -- Electrical Reference/LConn1
  voltage source 3/RConn2 -- Electrical Reference2/LConn1
  CLK/RConn1 -- voltage source 2/RConn1
  voltage source 2/RConn2 -- Electrical Reference1/LConn1
  B/RConn1 -- voltage source 3/RConn1
  A/RConn1 -- voltage source 1/RConn1

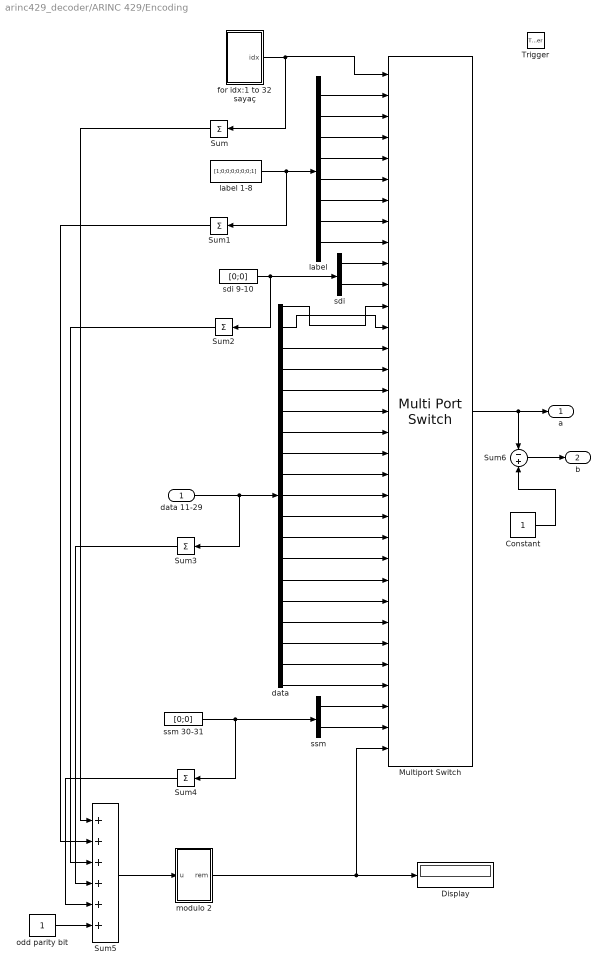
== system arinc429_decoder/ARINC 429/Encoding ==
  data 11-29 : Inport
  Trigger : TriggerPort  VariantControl=(inherit)
  Constant : Constant
  Display : Display
  Multiport Switch : MultiPortSwitch  Inputs=32  DiagnosticForDefault=None  InputSameDT=on
  Sum{,1..4} (5 alike) : Sum  Inputs=+
  Sum5 : Sum  Inputs=++++++
  Sum6 : Sum  Inputs=-+
  data : Demux  Outputs=19
  for idx:1 to 32 sayaç : Subsystem
  label : Demux  Outputs=8
  label 1-8 : Constant  Value=[1;0;0;0;0;0;0;1]  VectorParams1D=off
  modulo 2 : Subsystem
  odd parity bit : Constant
  sdi : Demux  Outputs=2
  sdi 9-10 : Constant  Value=[0;0]  VectorParams1D=off
  ssm : Demux  Outputs=2
  ssm 30-31 : Constant  Value=[0;0]  VectorParams1D=off
  a : Outport
  b : Outport  Port=2
  wires:
  for idx:1 to 32 sayaç/1(idx) -> Sum/1, Multiport Switch/1
  label/8 -> Multiport Switch/9
  label/7 -> Multiport Switch/8
  label/6 -> Multiport Switch/7
  label/5 -> Multiport Switch/6
  label/4 -> Multiport Switch/5
  label/3 -> Multiport Switch/4
  label/2 -> Multiport Switch/3
  label/1 -> Multiport Switch/2
  label 1-8/1 -> Sum1/1, label/1
  sdi/1 -> Multiport Switch/10
  sdi/2 -> Multiport Switch/11
  sdi 9-10/1 -> Sum2/1, sdi/1
  data/19 -> Multiport Switch/30
  data/18 -> Multiport Switch/29
  data/17 -> Multiport Switch/28
  data/16 -> Multiport Switch/27
  data/15 -> Multiport Switch/26
  data/14 -> Multiport Switch/25
  data/13 -> Multiport Switch/24
  data/12 -> Multiport Switch/23
  data/11 -> Multiport Switch/22
  data/10 -> Multiport Switch/21
  data/9 -> Multiport Switch/20
  data/8 -> Multiport Switch/19
  data/7 -> Multiport Switch/18
  data/6 -> Multiport Switch/17
  data/5 -> Multiport Switch/16
  data/4 -> Multiport Switch/15
  data/3 -> Multiport Switch/14
  data/2 -> Multiport Switch/13
  data/1 -> Multiport Switch/12
  data 11-29/1 -> Sum3/1, data/1
  ssm/1 -> Multiport Switch/31
  ssm/2 -> Multiport Switch/32
  ssm 30-31/1 -> Sum4/1, ssm/1
  Sum5/1 -> modulo 2/1(u)
  Sum/1 -> Sum5/1
  Sum1/1 -> Sum5/2
  Sum2/1 -> Sum5/3
  Sum3/1 -> Sum5/4
  Sum4/1 -> Sum5/5
  odd parity bit/1 -> Sum5/6
  Multiport Switch/1 -> Sum6/1, a/1
  Constant/1 -> Sum6/2
  Sum6/1 -> b/1
  modulo 2/1(rem) -> Display/1, Multiport Switch/33

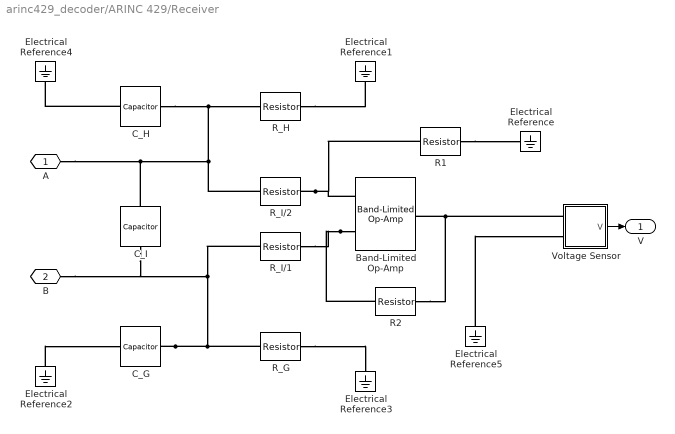
== system arinc429_decoder/ARINC 429/Receiver ==
  Band-Limited Op-Amp : ee_lib/Integrated Circuits/Band-Limited Op-Amp  A=1000  Rin=1e6 Ohm  Rout=100 Ohm  Vmin=-10 V  Vmax=10 V  Vdotmax=1e7 V/s  f=1e6 Hz  V0=0 V
      settings: SourceProductBaseCode=PS
  C_G : ee_lib/Passive/Capacitor  cap_option=0  c=50e-12 F  Cvec=[1e-05, 1e-06] F  Vvec=[0, 10] V  CV_table_symmetry=1  f_vec=[1, 10] kHz  DFext_vec=[.8, 1.2]  C_tol=0  enable_C_tol=0  tol_distribution=1  nSigma=4  r=1e-6 Ohm  g=0 1/Ohm  averaging_period=0 s  enable_operating_limits=0  operating_limit_action=2  max_working_voltage_range=[-25, 25] V  power_rating=1 W  enable_faults=0  fault_action=1  Cscale_faulted=100  R_faulted=1e-3 Ohm  G_faulted=0 1/Ohm  tau_fault=1e-3 s  enable_temporal_fault=0  t_fault=1 s  enable_behavioral_fault=0  max_permissible_voltage_range=[-100, 100] V  t_fail_on_voltage=1 s  i_specify=off  i_priority=None  i=0 A  i_nominal_specify=off  i_nominal_unit=A  i_nominal_value=1  v_specify=off  v_priority=None  v=0 V  v_nominal_specify=off  v_nominal_unit=V  v_nominal_value=1  vc_specify=off  vc_priority=High  vc=0 V  vc_nominal_specify=off  vc_nominal_unit=V  vc_nominal_value=1
  C_H : ee_lib/Passive/Capacitor  cap_option=0  c=50e-12 F  Cvec=[1e-05, 1e-06] F  Vvec=[0, 10] V  CV_table_symmetry=1  f_vec=[1, 10] kHz  DFext_vec=[.8, 1.2]  C_tol=0  enable_C_tol=0  tol_distribution=1  nSigma=4  r=1e-6 Ohm  g=0 1/Ohm  averaging_period=0 s  enable_operating_limits=0  operating_limit_action=2  max_working_voltage_range=[-25, 25] V  power_rating=1 W  enable_faults=0  fault_action=1  Cscale_faulted=100  R_faulted=1e-3 Ohm  G_faulted=0 1/Ohm  tau_fault=1e-3 s  enable_temporal_fault=0  t_fault=1 s  enable_behavioral_fault=0  max_permissible_voltage_range=[-100, 100] V  t_fail_on_voltage=1 s  i_specify=off  i_priority=None  i=0 A  i_nominal_specify=off  i_nominal_unit=A  i_nominal_value=1  v_specify=off  v_priority=None  v=0 V  v_nominal_specify=off  v_nominal_unit=V  v_nominal_value=1  vc_specify=off  vc_priority=High  vc=0 V  vc_nominal_specify=off  vc_nominal_unit=V  vc_nominal_value=1
  C_I : ee_lib/Passive/Capacitor  cap_option=0  c=50e-12 F  Cvec=[1e-05, 1e-06] F  Vvec=[0, 10] V  CV_table_symmetry=1  f_vec=[1, 10] kHz  DFext_vec=[.8, 1.2]  C_tol=0  enable_C_tol=0  tol_distribution=1  nSigma=4  r=1e-6 Ohm  g=0 1/Ohm  averaging_period=0 s  enable_operating_limits=0  operating_limit_action=2  max_working_voltage_range=[-25, 25] V  power_rating=1 W  enable_faults=0  fault_action=1  Cscale_faulted=100  R_faulted=1e-3 Ohm  G_faulted=0 1/Ohm  tau_fault=1e-3 s  enable_temporal_fault=0  t_fault=1 s  enable_behavioral_fault=0  max_permissible_voltage_range=[-100, 100] V  t_fail_on_voltage=1 s  i_specify=off  i_priority=None  i=0 A  i_nominal_specify=off  i_nominal_unit=A  i_nominal_value=1  v_specify=off  v_priority=None  v=0 V  v_nominal_specify=off  v_nominal_unit=V  v_nominal_value=1  vc_specify=off  vc_priority=High  vc=0 V  vc_nominal_specify=off  vc_nominal_unit=V  vc_nominal_value=1
  Electrical Reference{,1..5} (6 alike) : fl_lib/Electrical/Electrical Elements/Electrical Reference
  R1 : fl_lib/Electrical/Electrical Elements/Resistor  R=6 kOhm  i_specify=off  i_priority=None  i=0 A  i_nominal_specify=off  i_nominal_unit=A  i_nominal_value=1  v_specify=off  v_priority=None  v=0 V  v_nominal_specify=off  v_nominal_unit=V  v_nominal_value=1
  R2 : fl_lib/Electrical/Electrical Elements/Resistor  R=6 kOhm  i_specify=off  i_priority=None  i=0 A  i_nominal_specify=off  i_nominal_unit=A  i_nominal_value=1  v_specify=off  v_priority=None  v=0 V  v_nominal_specify=off  v_nominal_unit=V  v_nominal_value=1
  R_G : fl_lib/Electrical/Electrical Elements/Resistor  R=12 kOhm  i_specify=off  i_priority=None  i=0 A  i_nominal_specify=off  i_nominal_unit=A  i_nominal_value=1  v_specify=off  v_priority=None  v=0 V  v_nominal_specify=off  v_nominal_unit=V  v_nominal_value=1
  R_H : fl_lib/Electrical/Electrical Elements/Resistor  R=12 kOhm  i_specify=off  i_priority=None  i=0 A  i_nominal_specify=off  i_nominal_unit=A  i_nominal_value=1  v_specify=off  v_priority=None  v=0 V  v_nominal_specify=off  v_nominal_unit=V  v_nominal_value=1
  R_I/1 : fl_lib/Electrical/Electrical Elements/Resistor  R=12 kOhm  i_specify=off  i_priority=None  i=0 A  i_nominal_specify=off  i_nominal_unit=A  i_nominal_value=1  v_specify=off  v_priority=None  v=0 V  v_nominal_specify=off  v_nominal_unit=V  v_nominal_value=1
  R_I/2 : fl_lib/Electrical/Electrical Elements/Resistor  R=12 kOhm  i_specify=off  i_priority=None  i=0 A  i_nominal_specify=off  i_nominal_unit=A  i_nominal_value=1  v_specify=off  v_priority=None  v=0 V  v_nominal_specify=off  v_nominal_unit=V  v_nominal_value=1
  Voltage Sensor : Subsystem
  A : PMIOPort  Side=Left
  B : PMIOPort  Port=2  Side=Left
  V : Outport
  wires:
  Voltage Sensor/1(V) -> V/1
  connections:
  R1/RConn1 -- Electrical Reference/LConn1
  C_G/LConn1 -- R_G/LConn1 -- B/RConn1 -- C_I/RConn1 -- R_I/1/LConn1
  C_I/LConn1 -- A/RConn1 -- R_I/2/LConn1 -- C_H/LConn1 -- R_H/LConn1
  Band-Limited Op-Amp/LConn2 -- R_I/1/RConn1 -- R2/LConn1
  R_I/2/RConn1 -- R1/LConn1 -- Band-Limited Op-Amp/LConn1
  Electrical Reference2/LConn1 -- C_G/RConn1
  R_H/RConn1 -- Electrical Reference1/LConn1
  Electrical Reference5/LConn1 -- Voltage Sensor/LConn2
  R_G/RConn1 -- Electrical Reference3/LConn1
  C_H/RConn1 -- Electrical Reference4/LConn1
  R2/RConn1 -- Band-Limited Op-Amp/RConn1 -- Voltage Sensor/LConn1

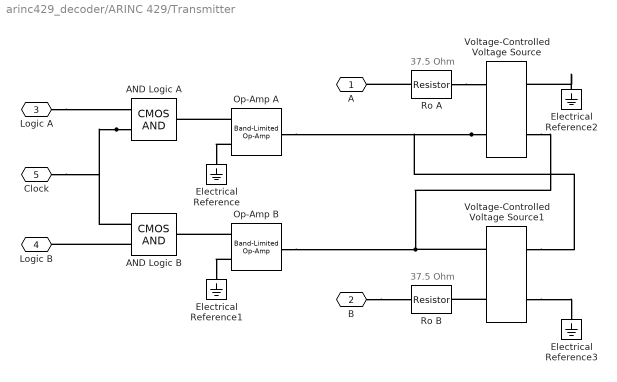
== system arinc429_decoder/ARINC 429/Transmitter ==
  note: 37.5 Ohm
  note: 37.5 Ohm
  " Op-Amp A" : ee_lib/Integrated Circuits/Band-Limited Op-Amp  A=1000  Rin=1e6 Ohm  Rout=37.5 Ohm  Vmin=-15 V  Vmax=15 V  Vdotmax=2e7 V/s  f=1e6 Hz  V0=0 V
      settings: SourceProductBaseCode=PS
  " Op-Amp B" : ee_lib/Integrated Circuits/Band-Limited Op-Amp  A=1000  Rin=1e6 Ohm  Rout=37.5 Ohm  Vmin=-10 V  Vmax=10 V  Vdotmax=2e7 V/s  f=1e6 Hz  V0=0 V
      settings: SourceProductBaseCode=PS
  AND Logic A : ee_lib/Integrated Circuits/Logic/CMOS AND  V_IL=0.1 V  V_IH=5 V  C_IN=5 pF  output_type=1  V_OL=0 V  V_OH=6.5 V  V_CC=5 V  V_meas=5 V  R_OUT=37.5 Ohm  R_OH=[25, 250] Ohm  I_OH=63 mA  R_OL=[30, 800] Ohm  I_OL=-45 mA  Delay=25 ns  Ron=5 Ohm  Vf=0.6 V  output_state=1
      settings: SourceProductBaseCode=PS  InternalSimscapePortConfiguration="{\"Bottom\":[],\"Left\":[{\"id\":\"A\",\"label\":\"\",\"type\":\"foundation.electrical.electrical\"},{\"id\":\"B\",\"label\":\"\",\"type\":\"foundation.electrical.electrical\"}],\"Right\":[{\"id\":\"J\",\"label\":\"\",\"type\":\"foundation.electrical.electrical\"}],\"Top\":[]}"
  AND Logic B : ee_lib/Integrated Circuits/Logic/CMOS AND  V_IL=0.1 V  V_IH=5 V  C_IN=5 pF  output_type=1  V_OL=0 V  V_OH=6.5 V  V_CC=5 V  V_meas=5 V  R_OUT=37.5 Ohm  R_OH=[25, 250] Ohm  I_OH=63 mA  R_OL=[30, 800] Ohm  I_OL=-45 mA  Delay=25 ns  Ron=5 Ohm  Vf=0.6 V  output_state=1
      settings: SourceProductBaseCode=PS  InternalSimscapePortConfiguration="{\"Bottom\":[],\"Left\":[{\"id\":\"A\",\"label\":\"\",\"type\":\"foundation.electrical.electrical\"},{\"id\":\"B\",\"label\":\"\",\"type\":\"foundation.electrical.electrical\"}],\"Right\":[{\"id\":\"J\",\"label\":\"\",\"type\":\"foundation.electrical.electrical\"}],\"Top\":[]}"
  Electrical Reference{,1..3} (4 alike) : fl_lib/Electrical/Electrical Elements/Electrical Reference
  Ro A : fl_lib/Electrical/Electrical Elements/Resistor  R=37.5 Ohm  i_specify=off  i_priority=None  i=0 A  i_nominal_specify=off  i_nominal_unit=A  i_nominal_value=1  v_specify=off  v_priority=None  v=0 V  v_nominal_specify=off  v_nominal_unit=V  v_nominal_value=1
  Ro B : fl_lib/Electrical/Electrical Elements/Resistor  R=37.5 Ohm  i_specify=off  i_priority=None  i=0 A  i_nominal_specify=off  i_nominal_unit=A  i_nominal_value=1  v_specify=off  v_priority=None  v=0 V  v_nominal_specify=off  v_nominal_unit=V  v_nominal_value=1
  Voltage-Controlled Voltage Source : fl_lib/Electrical/Electrical Sources/Voltage-Controlled Voltage Source  K=2.5  v1_specify=off  v1_priority=None  v1=0 V  v1_nominal_specify=off  v1_nominal_unit=V  v1_nominal_value=1  v2_specify=off  v2_priority=None  v2=0 V  v2_nominal_specify=off  v2_nominal_unit=V  v2_nominal_value=1
      settings: SourceProductBaseCode=SS  InternalSimscapePortConfiguration="{\"Bottom\":[],\"Left\":[{\"id\":\"p1\",\"label\":\"+\",\"type\":\"foundation.electrical.electrical\"},{\"id\":\"p2\",\"label\":\"+\",\"type\":\"foundation.electrical.electrical\"}],\"Right\":[{\"id\":\"n1\",\"label\":\"-\",\"type\":\"foundation.electrical.electrical\"},{\"id\":\"n2\",\"label\":\"-\",\"type\":\"foundation.electrical.electrical\"}],\"Top\":[]}"
  Voltage-Controlled Voltage Source1 : fl_lib/Electrical/Electrical Sources/Voltage-Controlled Voltage Source  K=2.5  v1_specify=off  v1_priority=None  v1=0 V  v1_nominal_specify=off  v1_nominal_unit=V  v1_nominal_value=1  v2_specify=off  v2_priority=None  v2=0 V  v2_nominal_specify=off  v2_nominal_unit=V  v2_nominal_value=1
      settings: SourceProductBaseCode=SS  InternalSimscapePortConfiguration="{\"Bottom\":[],\"Left\":[{\"id\":\"p1\",\"label\":\"+\",\"type\":\"foundation.electrical.electrical\"},{\"id\":\"p2\",\"label\":\"+\",\"type\":\"foundation.electrical.electrical\"}],\"Right\":[{\"id\":\"n1\",\"label\":\"-\",\"type\":\"foundation.electrical.electrical\"},{\"id\":\"n2\",\"label\":\"-\",\"type\":\"foundation.electrical.electrical\"}],\"Top\":[]}"
  A : PMIOPort  Side=Right
  B : PMIOPort  Port=2  Side=Right
  Logic A : PMIOPort  Port=3  Side=Left
  Logic B : PMIOPort  Port=4  Side=Left
  Clock : PMIOPort  Port=5  Side=Left
  connections:
  Voltage-Controlled Voltage Source/RConn1 -- " Op-Amp B"/RConn1 -- Voltage-Controlled Voltage Source1/LConn1
  Voltage-Controlled Voltage Source/LConn1 -- " Op-Amp A"/RConn1 -- Voltage-Controlled Voltage Source1/RConn1
  AND Logic A/LConn2 -- Clock/RConn1 -- AND Logic B/LConn1
  " Op-Amp A"/LConn1 -- AND Logic A/RConn1
  " Op-Amp B"/LConn1 -- AND Logic B/RConn1
  Electrical Reference2/LConn1 -- Voltage-Controlled Voltage Source/RConn2
  AND Logic B/LConn2 -- Logic B/RConn1
  Ro A/LConn1 -- Voltage-Controlled Voltage Source/LConn2
  " Op-Amp A"/LConn2 -- Electrical Reference/LConn1
  Voltage-Controlled Voltage Source1/RConn2 -- Electrical Reference3/LConn1
  Ro A/RConn1 -- A/RConn1
  Logic A/RConn1 -- AND Logic A/LConn1
  " Op-Amp B"/LConn2 -- Electrical Reference1/LConn1
  Voltage-Controlled Voltage Source1/LConn2 -- Ro B/LConn1
  B/RConn1 -- Ro B/RConn1

== system arinc429_decoder/ARINC 429/decoder  ==
  rx : Inport
  Trigger : TriggerPort  VariantControl=(inherit)
  Constant : Constant  Value=5
  Constant1 : Constant  Value=-5
  Constant2 : Constant  Value=0
  Relational Operator : RelationalOperator  Operator=>  OutDataTypeStr=boolean  RndMeth=Simplest
  Relational Operator1 : RelationalOperator  Operator=<  OutDataTypeStr=boolean  RndMeth=Simplest
  Switch : Switch  Criteria=u2 ~= 0
  Outport : Outport
  wires:
  Constant1/1 -> Relational Operator1/1
  Constant/1 -> Relational Operator/1
  Constant2/1 -> Switch/2
  Relational Operator1/1 -> Switch/3
  Relational Operator/1 -> Switch/1
  Switch/1 -> Outport/1
  rx/1 -> Relational Operator1/2, Relational Operator/2

== system arinc429_decoder/ARINC 1/DAC/voltage source 1 ==
  S : Inport
  Controlled Voltage Source : fl_lib/Electrical/Electrical Sources/Controlled Voltage Source
  Gain : Gain  Gain=5  SaturateOnIntegerOverflow=on  ParamDataTypeStr=Inherit: Same as input
  Simulink-PS Converter1 : nesl_utility/Simulink-PS Converter  PhysicalDomain=network_engine_domain  SubClassName=ps_input  LeftPortType=input  RightPortType=output  PseudoPeriodic=off  Frequencies=[]  NoiseDistribution=none  NoiseParameters=[]  Unit=1  AffineConversion=off  FilteringAndDerivatives=filter  SimscapeFilterOrder=1  InputFilterTimeConstant=1.5e-6  UdotUserProvided=0
      settings: SourceProductBaseCode=PW,SS
  Solver Configuration : nesl_utility/Solver Configuration  PhysicalDomain=network_engine_domain  SubClassName=solver  LeftPortType=input  RightPortType=generic  Tones=[]  Harmonics=[]  SimulateNoise=off  Profile=off  UseLocalSampling=off  EnableSwitchedLinearOptims=on  FrequencyDomain=off  UseCCode=off  RelTol=0.001  AbsTol=1e-06  MinStep=1e-09  ToWorkspace=off  RevertToSquareIcSolve=off  NumHomotopyIterations=100  PhasorMode=off  PhasorModeNumHarmonics=1  DoDC=off  ResidualTolerance=1e-09  UseLocalSolver=off  LocalSolverChoice=NE_BACKWARD_EULER_ADVANCER  LocalSolverSampleTime=0.001  DoFixedCost=off  MaxNonlinIter=3  MaxModeIter=2  ComputeImpulses=off  ImpulseIterations=2  LinearAlgebra=auto  EquationFormulation=NE_TIME_EF  DelaysMemoryBudget=1024  AutomaticFiltering=on  FilteringTimeConstant=0.001  PartitionStorageMethod=AS_NEEDED  PartitionMemoryBudget=1024  PartitionMethod=ROBUST
      settings: SourceProductBaseCode=PW,SS
  + : PMIOPort  Side=Right
  - : PMIOPort  Port=2  Side=Right
  wires:
  S/1 -> Gain/1
  Gain/1 -> Simulink-PS Converter1/1
  connections:
  Solver Configuration/RConn1 -- Simulink-PS Converter1/RConn1 -- Controlled Voltage Source/RConn1
  -/RConn1 -- Controlled Voltage Source/RConn2
  +/RConn1 -- Controlled Voltage Source/LConn1

== system arinc429_decoder/ARINC 1/DAC/voltage source 2 ==
  S : Inport
  Controlled Voltage Source : fl_lib/Electrical/Electrical Sources/Controlled Voltage Source
  Gain : Gain  Gain=5  SaturateOnIntegerOverflow=on  ParamDataTypeStr=Inherit: Same as input
  Simulink-PS Converter : nesl_utility/Simulink-PS Converter  PhysicalDomain=network_engine_domain  SubClassName=ps_input  LeftPortType=input  RightPortType=output  PseudoPeriodic=off  Frequencies=[]  NoiseDistribution=none  NoiseParameters=[]  Unit=1  AffineConversion=off  FilteringAndDerivatives=filter  SimscapeFilterOrder=1  InputFilterTimeConstant=1.5e-6  UdotUserProvided=0
      settings: SourceProductBaseCode=PW,SS
  + : PMIOPort  Side=Right
  - : PMIOPort  Port=2  Side=Right
  wires:
  S/1 -> Gain/1
  Gain/1 -> Simulink-PS Converter/1
  connections:
  Simulink-PS Converter/RConn1 -- Controlled Voltage Source/RConn1
  -/RConn1 -- Controlled Voltage Source/RConn2
  +/RConn1 -- Controlled Voltage Source/LConn1

== system arinc429_decoder/ARINC 1/DAC/voltage source 3 ==
  S : Inport
  Controlled Voltage Source : fl_lib/Electrical/Electrical Sources/Controlled Voltage Source
  Gain : Gain  Gain=5  SaturateOnIntegerOverflow=on  ParamDataTypeStr=Inherit: Same as input
  Simulink-PS Converter : nesl_utility/Simulink-PS Converter  PhysicalDomain=network_engine_domain  SubClassName=ps_input  LeftPortType=input  RightPortType=output  PseudoPeriodic=off  Frequencies=[]  NoiseDistribution=none  NoiseParameters=[]  Unit=1  AffineConversion=off  FilteringAndDerivatives=filter  SimscapeFilterOrder=1  InputFilterTimeConstant=1.5e-6  UdotUserProvided=0
      settings: SourceProductBaseCode=PW,SS
  + : PMIOPort  Side=Right
  - : PMIOPort  Port=2  Side=Right
  wires:
  S/1 -> Gain/1
  Gain/1 -> Simulink-PS Converter/1
  connections:
  Simulink-PS Converter/RConn1 -- Controlled Voltage Source/RConn1
  -/RConn1 -- Controlled Voltage Source/RConn2
  +/RConn1 -- Controlled Voltage Source/LConn1

== system arinc429_decoder/ARINC 1/Encoding/for idx:1 to 32 sayaç ==
  Constant : Constant
  Scope : Scope
  Sum : Sum  Inputs=|++  InputSameDT=on  SaturateOnIntegerOverflow=on
  Unit Delay : UnitDelay  InitialCondition=1  SampleTime=-1  HasFrameUpgradeWarning=on
  idx : Outport
  wires:
  Unit Delay/1 -> Sum/2, idx/1, Scope/1
  Constant/1 -> Sum/1
  Sum/1 -> Unit Delay/1

== system arinc429_decoder/ARINC 1/Encoding/modulo 2 ==
  u : Inport
  Constant : Constant  Value=2
  Math Function : Math  Operator=rem  SaturateOnIntegerOverflow=on
  Sum : Sum  Inputs=+
  rem : Outport
  wires:
  u/1 -> Sum/1
  Sum/1 -> Math Function/1
  Constant/1 -> Math Function/2
  Math Function/1 -> rem/1
